simulink library "csc_tcs_thermal_control_system_lib"  (R2014b)
settings: Solver=ode113  StartTime=0.0  StopTime=10.0  RelTol=1e-3
undefined symbols (not defined in the file or in its folder): fsw_dt
libraries: util_common_lib x2, util_info_lib x1, csu_cmt_convert_measured_temps_collection_lib x1, csu_cmx_convert_measured_pressure_xducer_collection_lib x1
settings Model: Creator=Jim Kaidy  LastModifiedBy=mstewart

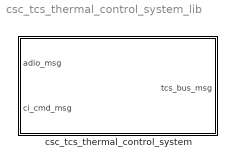
== system csc_tcs_thermal_control_system_lib ==
  csc_tcs_thermal_control_system : Subsystem  Tag=OFSW; MDL_TICK=ADIO_MSG  TreatAsAtomicUnit=on  SystemSampleTime=fsw_dt

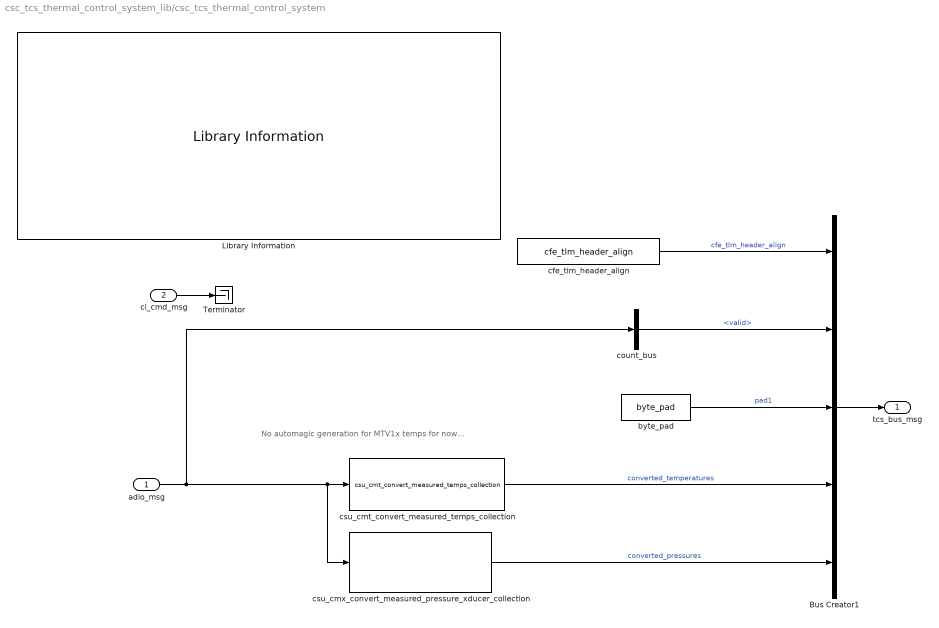
== system csc_tcs_thermal_control_system_lib/csc_tcs_thermal_control_system ==
  note: No automagic generation for MTV1x temps for now...
  adio_msg : Inport
  ci_cmd_msg : Inport  Port=2
  Bus Creator1 : BusCreator  Inputs=5  OutDataTypeStr=Bus: tcs_bus_msg  NonVirtualBus=on
  Library Information : util_info_lib/Library Information  owner='escrane'
  Terminator : Terminator
  byte_pad : util_common_lib/byte_pad  n_bytes=7
  cfe_tlm_header_align : util_common_lib/cfe_tlm_header_align
  count_bus : BusSelector  OutputSignals=valid
  csu_cmt_convert_measured_temps_collection : csu_cmt_convert_measured_temps_collection_lib/csu_cmt_convert_measured_temps_collection
  csu_cmx_convert_measured_pressure_xducer_collection : csu_cmx_convert_measured_pressure_xducer_collection_lib/csu_cmx_convert_measured_pressure_xducer_collection  SystemSampleTime=-1
  tcs_bus_msg : Outport  OutDataTypeStr=Bus: tcs_bus_msg
  wires:
  byte_pad/1 -> Bus Creator1/3  "pad1"
  count_bus/1 -> Bus Creator1/2  "<valid>"
  cfe_tlm_header_align/1 -> Bus Creator1/1  "cfe_tlm_header_align"
  ci_cmd_msg/1 -> Terminator/1
  Bus Creator1/1 -> tcs_bus_msg/1
  adio_msg/1 -> csu_cmx_convert_measured_pressure_xducer_collection/1, csu_cmt_convert_measured_temps_collection/1, count_bus/1
  csu_cmt_convert_measured_temps_collection/1 -> Bus Creator1/4  "converted_temperatures"
  csu_cmx_convert_measured_pressure_xducer_collection/1 -> Bus Creator1/5  "converted_pressures"
